simulink model "launchpad_R2012a"  (Simulink 7.9)
settings: Solver=FixedStepDiscrete  StartTime=0.0  StopTime=10  FixedStep=0.1  RelTol=1e-3
PreLoadFcn:
  | use_hardware = 0;
  | hardware_variant = Simulink.Variant('use_hardware == 1');
  | software_variant = Simulink.Variant('use_hardware == 0');
undefined symbols (not defined in the file or in its folder): sigbuilder_block
libraries: launchpad_lib x4, simulink x1
settings Model: Creator=bas  LastModifiedBy=peselnikmg
settings OptimizationCC: OptimizeModelRefInitCode=on  LifeSpan=Inf
settings HardwareCC: ProdBitPerInt=16  ProdBitPerPointer=16  ProdIntDivRoundTo=Zero  ProdEndianess=LittleEndian  ProdWordSize=16  ProdHWDeviceType=Texas Instruments->MSP430
settings RTWCC: SystemTargetFile=launchpad.tlc  TemplateMakefile=launchpad_tmf  Description=TI LaunchPad  GenerateReport=on  ProcessScript=launchpad_make_rtw_hook  IncludeHyperlinkInReport=on  GenerateTraceInfo=on  GenerateTraceReport=on  GenerateTraceReportSl=on  GenerateTraceReportSf=on  GenerateTraceReportEml=on
settings CodeAppCC: IgnoreCustomStorageClasses=off
settings STFCustomTargetCC: CodeReplacementLibrary=ANSI_C  CombineOutputUpdateFcns=on  ERTCustomFileBanners=on  SupportContinuousTime=off  SupportNonInlinedSFcns=off  GRTInterface=off  SystemTargetFile=launchpad.tlc
settings ERTTargetCC: CodeReplacementLibrary=ANSI_C  MultiwordLength=2048  ParMdlRefBuildCompliant=off  CompOptLevelCompliant=off  ConcurrentExecutionCompliant=off  ERTFirstTimeCompliant=off  ModelStepFunctionPrototypeControlCompliant=off  CPPClassGenCompliant=off  ExtModeMexFile=noextcomm  InlinedParameterPlacement=NonHierarchical  ERTCustomFileTemplate=launchpad_srmain.tlc  ConvertIfToSwitch=off  SuppressUnreachableDefaultCases=off
settings CustomProperty: Value=on

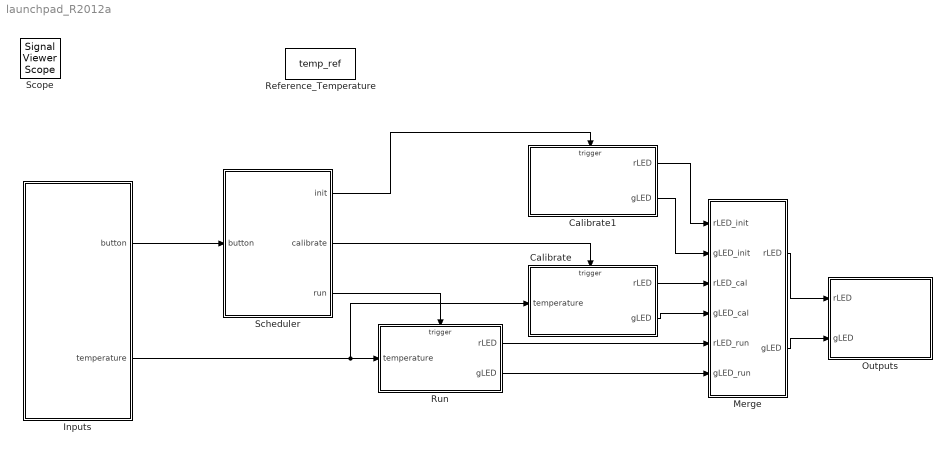
== system launchpad_R2012a ==
  Calibrate : Subsystem
  Calibrate1 : Subsystem
  Inputs : Subsystem  Variant=on
  Merge : Subsystem
  Outputs : Subsystem  Variant=on
  Reference_Temperature : DataStoreMemory  DataStoreName=temp_ref  ReadBeforeWriteMsg=warning  WriteAfterWriteMsg=warning  WriteAfterReadMsg=warning  OutDataTypeStr=uint8
  Run : Subsystem
  Scheduler : Subsystem
  Scope : SignalViewerScope  IOType=viewer  RefreshTime=0.035000
  wires:
  Scheduler/2(calibrate) -> Calibrate/Trigger
  Scheduler/3(run) -> Run/Trigger
  Inputs/1(button) -> Scheduler/1(button)
  Merge/1(rLED) -> Outputs/1(rLED)
  Merge/2(gLED) -> Outputs/2(gLED)
  Calibrate/1(rLED) -> Merge/3(rLED_cal)
  Calibrate/2(gLED) -> Merge/4(gLED_cal)
  Run/1(rLED) -> Merge/5(rLED_run)
  Run/2(gLED) -> Merge/6(gLED_run)
  Inputs/2(temperature) -> Run/1(temperature), Calibrate/1(temperature)
  Scheduler/1(init) -> Calibrate1/Trigger
  Calibrate1/1(rLED) -> Merge/1(rLED_init)
  Calibrate1/2(gLED) -> Merge/2(gLED_init)

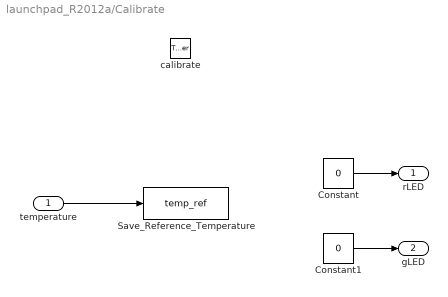
== system launchpad_R2012a/Calibrate ==
  temperature : Inport
  calibrate : TriggerPort  TriggerType=function-call  PortDimensions=1
  Constant : Constant  Value=0  OutDataTypeStr=uint8
  Constant1 : Constant  Value=0  OutDataTypeStr=uint8
  Save_Reference_Temperature : DataStoreWrite  DataStoreName=temp_ref
  rLED : Outport  InitialOutput=0
  gLED : Outport  Port=2  InitialOutput=0
  wires:
  Constant/1 -> rLED/1
  Constant1/1 -> gLED/1
  temperature/1 -> Save_Reference_Temperature/1

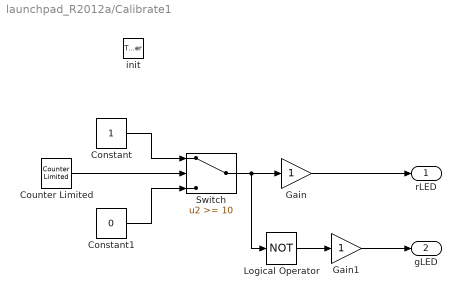
== system launchpad_R2012a/Calibrate1 ==
  init : TriggerPort  TriggerType=function-call  PortDimensions=1
  Constant : Constant  OutDataTypeStr=uint8
  Constant1 : Constant  Value=0  OutDataTypeStr=uint8
  Counter Limited : simulink/Sources/Counter Limited  uplimit=19  tsamp=-1
      settings: AttributesFormatString=Limit=%<uplimit>
  Gain : Gain  OutDataTypeStr=uint8
  Gain1 : Gain  OutDataTypeStr=uint8
  Logical Operator : Logic  Operator=NOT  AllPortsSameDT=off  OutDataTypeStr=boolean
  Switch : Switch  Threshold=10
      settings: AttributesFormatString=Threshold=%<Threshold>
  rLED : Outport
  gLED : Outport  Port=2
  wires:
  Gain/1 -> rLED/1
  Logical Operator/1 -> Gain1/1
  Counter Limited/1 -> Switch/2
  Constant1/1 -> Switch/3
  Constant/1 -> Switch/1
  Switch/1 -> Gain/1, Logical Operator/1
  Gain1/1 -> gLED/1

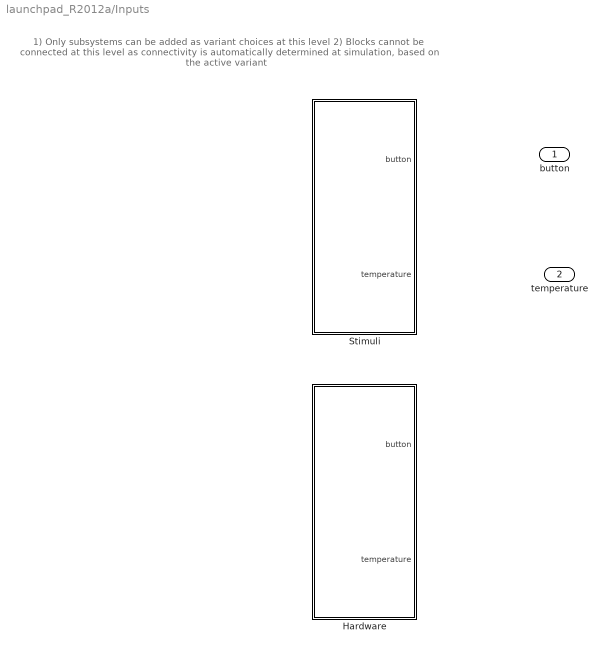
== system launchpad_R2012a/Inputs ==
  note: 1) Only subsystems can be added as variant choices at this level
      | 2) Blocks cannot be connected at this level as connectivity is
      | automatically determined at simulation, based on the active variant
  Hardware : Subsystem  VariantObject=hardware_variant
  Stimuli : Subsystem  VariantObject=software_variant
  button : Outport
  temperature : Outport  Port=2

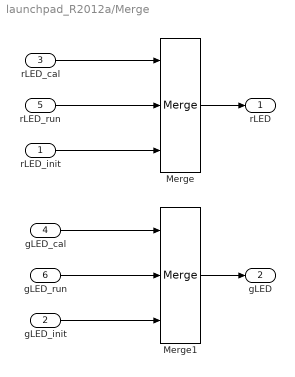
== system launchpad_R2012a/Merge ==
  rLED_init : Inport
  gLED_init : Inport  Port=2
  rLED_cal : Inport  Port=3
  gLED_cal : Inport  Port=4
  rLED_run : Inport  Port=5
  gLED_run : Inport  Port=6
  Merge : Merge  Inputs=3
  Merge1 : Merge  Inputs=3
  rLED : Outport
  gLED : Outport  Port=2
  wires:
  rLED_cal/1 -> Merge/1
  Merge/1 -> rLED/1
  rLED_run/1 -> Merge/2
  gLED_cal/1 -> Merge1/1
  Merge1/1 -> gLED/1
  gLED_run/1 -> Merge1/2
  rLED_init/1 -> Merge/3
  gLED_init/1 -> Merge1/3

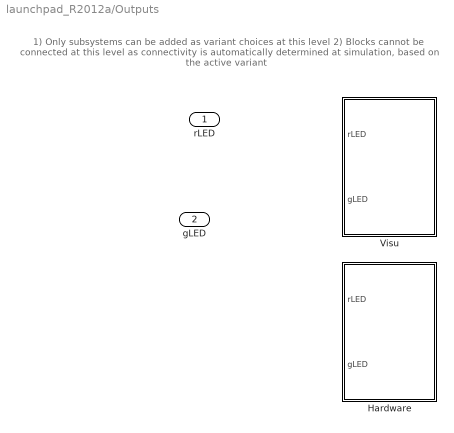
== system launchpad_R2012a/Outputs ==
  note: 1) Only subsystems can be added as variant choices at this level
      | 2) Blocks cannot be connected at this level as connectivity is
      | automatically determined at simulation, based on the active variant
  rLED : Inport
  gLED : Inport  Port=2
  Hardware : Subsystem  VariantObject=hardware_variant
  Visu : Subsystem  VariantObject=software_variant

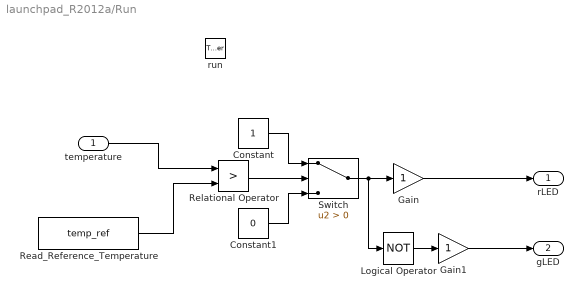
== system launchpad_R2012a/Run ==
  temperature : Inport
  run : TriggerPort  TriggerType=function-call  PortDimensions=1
  Constant : Constant  OutDataTypeStr=uint8
  Constant1 : Constant  Value=0  OutDataTypeStr=uint8
  Gain : Gain  OutDataTypeStr=uint8
  Gain1 : Gain  OutDataTypeStr=uint8
  Logical Operator : Logic  Operator=NOT  AllPortsSameDT=off  OutDataTypeStr=boolean
  Read_Reference_Temperature : DataStoreRead  DataStoreName=temp_ref
  Relational Operator : RelationalOperator  Operator=>  OutDataTypeStr=boolean
  Switch : Switch  Criteria=u2 > Threshold
  rLED : Outport
  gLED : Outport  Port=2
  wires:
  temperature/1 -> Relational Operator/1
  Read_Reference_Temperature/1 -> Relational Operator/2
  Relational Operator/1 -> Switch/2
  Switch/1 -> Logical Operator/1, Gain/1
  Logical Operator/1 -> Gain1/1
  Constant/1 -> Switch/1
  Constant1/1 -> Switch/3
  Gain/1 -> rLED/1
  Gain1/1 -> gLED/1

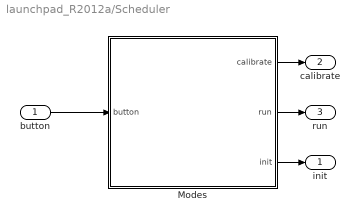
== system launchpad_R2012a/Scheduler ==
  button : Inport
  Modes : Stateflow chart  TreatAsAtomicUnit=on
  init : Outport
  calibrate : Outport  Port=2
  run : Outport  Port=3
  wires:
  Modes/1(calibrate) -> calibrate/1
  Modes/2(run) -> run/1
  button/1 -> Modes/1(button)
  Modes/3(init) -> init/1

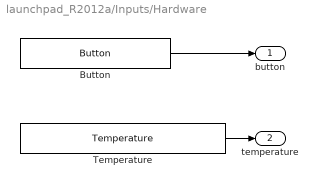
== system launchpad_R2012a/Inputs/Hardware ==
  Button : launchpad_lib/Button  SFunctionSpec=uint8 y1 = button_get(void)  ShowSpec=on
  Temperature : launchpad_lib/Temperature  SFunctionSpec=uint8 y1 = temperature_read(uint8 p1)  SParameter1=Celsius  ShowSpec=on
      settings: AttributesFormatString=%<SParameter1>
  button : Outport  OutDataTypeStr=uint8
  temperature : Outport  Port=2  OutDataTypeStr=uint8
  wires:
  Temperature/1 -> temperature/1
  Button/1 -> button/1

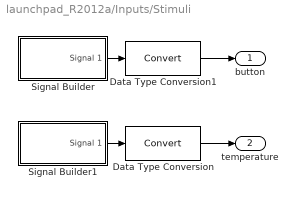
== system launchpad_R2012a/Inputs/Stimuli ==
  Data Type Conversion : DataTypeConversion
  Data Type Conversion1 : DataTypeConversion
  Signal Builder : Subsystem  Tag=STV Subsys  LoadFcn=sigbuilder_block('load');  StartFcn=sigbuilder_block('start');  StopFcn=sigbuilder_block('stop');  ClipboardFcn=sigbuilder_block('clipboard');  mask(Sigbuilder block){}
      mask help: Simulink:masks:SigbuilderBlock_MD
      mask init:
      | if ~strcmp(get_param(bdroot(gcbh),'SimulationStatus'),'stopped') tuvar = sigbuilder_block('maskInit'); end
      settings: CopyFcn=sigbuilder_block('copy');  DeleteFcn=sigbuilder_block('delete');  ModelCloseFcn=sigbuilder_block('modelClose');  PreSaveFcn=sigbuilder_block('preSave');  PauseFcn=sigbuilder_block('pause');  ContinueFcn=sigbuilder_block('continue');  NameChangeFcn=sigbuilder_block('namechange');  OpenFcn=sigbuilder_block('open',[99 153 550.5 399.75 ]);  CloseFcn=sigbuilder_block('close');
      mask Display: plot(0, 0, 100, 100,[2, 2, 32, 32, 2], [68, 8, 8, 68, 68],[32, 2], [38, 38], [32, 19, 2],[53, 60, 44], [32, 17, 17, 2],[16, 16, 31, 31]);txt = getActiveGroup(gcbh);text(2, 100, txt,'verticalAlignment', 'top');
  Signal Builder1 : Subsystem  Tag=STV Subsys  LoadFcn=sigbuilder_block('load');  StartFcn=sigbuilder_block('start');  StopFcn=sigbuilder_block('stop');  ClipboardFcn=sigbuilder_block('clipboard');  mask(Sigbuilder block){}
      mask help: Simulink:masks:SigbuilderBlock_MD
      mask init:
      | if ~strcmp(get_param(bdroot(gcbh),'SimulationStatus'),'stopped') tuvar = sigbuilder_block('maskInit'); end
      settings: CopyFcn=sigbuilder_block('copy');  DeleteFcn=sigbuilder_block('delete');  ModelCloseFcn=sigbuilder_block('modelClose');  PreSaveFcn=sigbuilder_block('preSave');  PauseFcn=sigbuilder_block('pause');  ContinueFcn=sigbuilder_block('continue');  NameChangeFcn=sigbuilder_block('namechange');  OpenFcn=sigbuilder_block('open',[437.25 199.5 550.5 399.75 ]);  CloseFcn=sigbuilder_block('close');
      mask Display: plot(0, 0, 100, 100,[2, 2, 32, 32, 2], [68, 8, 8, 68, 68],[32, 2], [38, 38], [32, 19, 2],[53, 60, 44], [32, 17, 17, 2],[16, 16, 31, 31]);txt = getActiveGroup(gcbh);text(2, 100, txt,'verticalAlignment', 'top');
  button : Outport  OutDataTypeStr=uint8
  temperature : Outport  Port=2  OutDataTypeStr=uint8
  wires:
  Data Type Conversion1/1 -> button/1
  Data Type Conversion/1 -> temperature/1
  Signal Builder1/1(Signal 1) -> Data Type Conversion/1
  Signal Builder/1(Signal 1) -> Data Type Conversion1/1

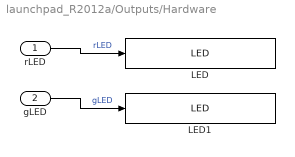
== system launchpad_R2012a/Outputs/Hardware ==
  rLED : Inport
  gLED : Inport  Port=2
  LED : launchpad_lib/LED  SFunctionSpec=led_set(uint8 p1, uint8 u1)  SParameter1=Red  ShowSpec=on
      settings: AttributesFormatString=LED: %<SParameter1>
  LED1 : launchpad_lib/LED  SFunctionSpec=led_set(uint8 p1, uint8 u1)  SParameter1=Green  ShowSpec=on
      settings: AttributesFormatString=LED: %<SParameter1>
  wires:
  rLED/1 -> LED/1  "rLED"
  gLED/1 -> LED1/1  "gLED"

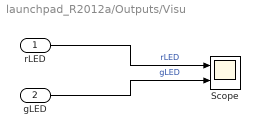
== system launchpad_R2012a/Outputs/Visu ==
  rLED : Inport
  gLED : Inport  Port=2
  Scope : Scope  NumInputPorts=2
      settings: YMin=-5~-5  YMax=5~5
  wires:
  rLED/1 -> Scope/1  "rLED"
  gLED/1 -> Scope/2  "gLED"

== system launchpad_R2012a/Inputs/Stimuli/Signal Builder ==
  Demux : Demux  Tag=STV Demux  Outputs=1
  FromWs : FromWorkspace  Tag=STV FromWs  VariableName=tuvar  SampleTime=0  SigBuilderData=DataTag0  VnvData=DataTag1
      SigBuilderData=|
      | common.afterFinalStr = 'Extrapolate'
      | common.sampleTime = 0
      | dataSet.timeRange = [0 10]
      | dataSet.name = 'Group 1'
      | sbobj.Groups.Name = 'Group 1'
      | sbobj.Groups.Signals.Name = 'Signal 1'
      | sbobj.Groups.Signals.XData = [0 3 3 3.1 3.1 7 7 7.1 7.1 10]
      | sbobj.Groups.Signals.YData = [0 0 1 1 0 0 1 1 0 0]
  Signal 1 : Outport  Tag=STV Outport
  wires:
  FromWs/1 -> Demux/1
  Demux/1 -> Signal 1/1

== system launchpad_R2012a/Inputs/Stimuli/Signal Builder1 ==
  Demux : Demux  Tag=STV Demux  Outputs=1
  FromWs : FromWorkspace  Tag=STV FromWs  VariableName=tuvar  SampleTime=0  SigBuilderData=DataTag2  VnvData=DataTag3
      SigBuilderData=|
      | common.afterFinalStr = 'Extrapolate'
      | common.sampleTime = 0
      | dataSet.timeRange = [0 10]
      | dataSet.name = 'Group 1'
      | sbobj.Groups.Name = 'Group 1'
      | sbobj.Groups.Signals.Name = 'Signal 1'
      | sbobj.Groups.Signals.XData = [0 5 6.28 10]
      | sbobj.Groups.Signals.YData = [0 110 35.5 0]
  Signal 1 : Outport  Tag=STV Outport
  wires:
  Demux/1 -> Signal 1/1
  FromWs/1 -> Demux/1

== stateflow chart Scheduler/Modes ==
  state Calibrate
    en:calibrate;
  state Run
    du:run;
  state Init
    du:init;
  (default) -> Init
  Init -> Calibrate : [button > 0]
  Calibrate -> Run
  Run -> Calibrate : [button > 0]
  data: button input double
  events: calibrate output FUNCTION_CALL_EVENT; run output FUNCTION_CALL_EVENT; init output FUNCTION_CALL_EVENT
